simulink model "UpperLimb_ForwardDynamics"  (R2024b)
settings: Solver=VariableStepAuto  StartTime=0.0  StopTime=10.0  RelTol=1e-3
undefined symbols (not defined in the file or in its folder): b12, b23, g, I2S2, I3S3, L2, LS2, LS3, m2, m3
settings Model: Creator=jakub  LastModifiedBy=jakub

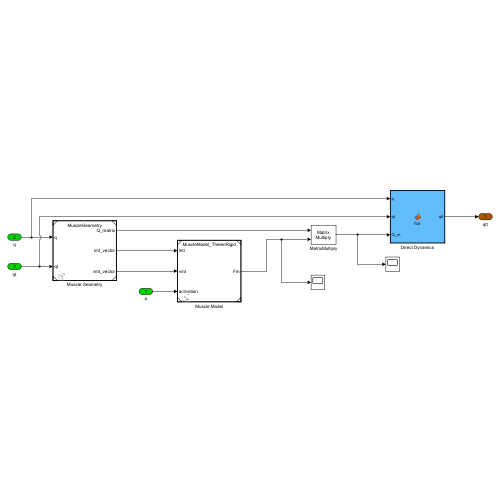
[thumbnail: Simulink's stored preview of the top-level diagram]
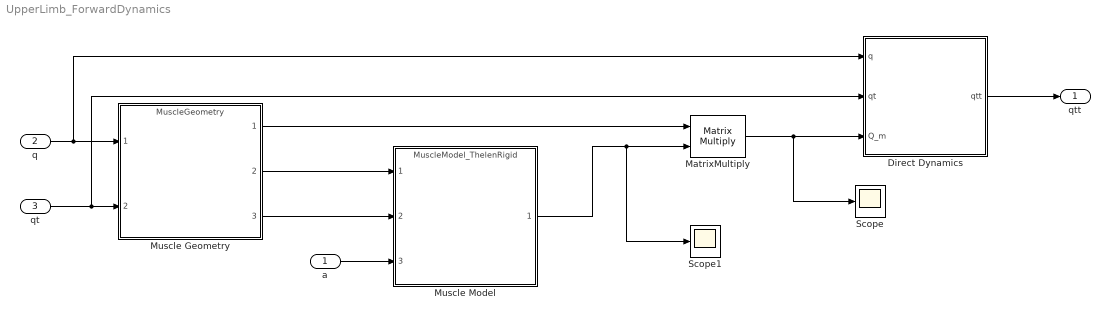
== system UpperLimb_ForwardDynamics ==
  a : Inport  OutMin=0  OutMax=1  OutDataTypeStr=double  PortDimensions=[8 1]  SampleTime=0
  q : Inport  Port=2  OutDataTypeStr=double  Unit=rad  PortDimensions=[2 1]  SampleTime=0
  qt : Inport  Port=3  OutDataTypeStr=double  Unit=rad/sec  PortDimensions=[2 1]  SampleTime=0
  Direct Dynamics : MATLAB Function  TreatAsAtomicUnit=on
  MatrixMultiply : Product  Multiplication=Matrix(*)  OutDataTypeStr=double
  Muscle Geometry : ModelReference  ModelNameDialog=MuscleGeometry.slx  SimulationMode=Normal  ModelReferenceVersion=1.156
  Muscle Model : ModelReference  ModelNameDialog=MuscleModel_ThelenRigid.slx  SimulationMode=Normal  ModelReferenceVersion=1.25
  Scope : Scope
  Scope1 : Scope
  qtt : Outport  OutDataTypeStr=double  Unit=rad/s^2  PortDimensions=[2 1]  SampleTime=0
  wires:
  a/1 -> Muscle Model/3
  Muscle Model/1 -> Scope1/1, MatrixMultiply/2
  Muscle Geometry/2 -> Muscle Model/1
  Muscle Geometry/1 -> MatrixMultiply/1
  Muscle Geometry/3 -> Muscle Model/2
  MatrixMultiply/1 -> Scope/1, Direct Dynamics/3(Q_m)
  Direct Dynamics/1(qtt) -> qtt/1
  q/1 -> Direct Dynamics/1(q), Muscle Geometry/1
  qt/1 -> Direct Dynamics/2(qt), Muscle Geometry/2

== matlab function UpperLimb_ForwardDynamics/Direct Dynamics ==
  data: q input double size=[2 1]; qtt output double size=[2 1]; qt input double size=[2 1]; Q_m input double size=[2 1]; m2 parameter double size=1; m3 parameter double size=1; L2 parameter double size=1; LS2 parameter double size=1; LS3 parameter double size=1; g parameter double size=1; I2S2 parameter double size=1; I3S3 parameter double size=1; b12 parameter double size=1; b23 parameter double size=1
function qtt = fcn(q, qt, Q_m, m2, m3, L2, LS2, LS3, g, I2S2, I3S3, b12, b23)
    G2 = m2*g; G3 = m3*g;

% position, velocity
    fi12 = q(1); fi13 = q(2);
    fi12t = qt(1); fi13t = qt(2);



% Mass Matrix
M = [m2*LS2^2 + I2S2 + m3*L2^2, m3*L2*LS3*cos(fi12 - fi13);
     m3*L2*LS3*cos(fi12 - fi13), m3*LS3^2 + I3S3];

% Corriolis and other acc
H = [fi13t^2*m3*L2*LS3*sin(fi12-fi13);
     -fi12t^2*m3*L2*LS3*sin(fi12-fi13)];

% Gravity forces
Q_g = [-G2*LS2*cos(fi12) - G3*L2*cos(fi12); - G3*LS3*cos(fi13)];

% Damping
Q_b = [-b12*fi12t + b23*(fi13t-fi12t);
       -b23*(fi13t-fi12t)];

Q = Q_g + Q_m + Q_b;

qtt = M\(Q - H);
